simulink model "Vehicle_Model"  (R2018b)
settings: Solver=VariableStepAuto  StartTime=0  StopTime=60  FixedStep=0.0000001  RelTol=1e-10
undefined symbols (not defined in the file or in its folder): Initial
(part 4 of 4)

== matlab function Vehicle_Model/Subsystem3/MATLAB Function8 ==
  data: Fz input; Fxo output; kappa input; alpha input; gam input; Fzo input; Ro input; q_Bz1 input; q_Bz2 input; q_Bz3 input; q_Bz4 input; q_Bz5 input; q_Bz9 input; q_Bz10 input; q_Cz1 input; q_Dz1 input; q_Dz2 input; q_Dz3 input; q_Dz4 input; q_Dz6 input; q_Dz7 input; q_Dz8 input; q_Dz9 input; q_Ez1 input; q_Ez2 input; q_Ez3 input; q_Ez4 input; q_Ez5 input; q_Hz1 input; q_Hz2 input; q_Hz3 input; q_Hz4 input; p_Cy1 input; p_Dy1 input; p_Dy2 input; p_Dy3 input; p_Ey1 input; p_Ey2 input; p_Ey3 input; p_Ey4 input; p_Ky1 input; p_Ky2 input; p_Ky3 input; p_Hy1 input; p_Hy2 input; p_Hy3 input; p_Vy1 input; p_Vy2 input; p_Vy3 input; p_Vy4 input; p_Cx1 input; p_Dx1 input; p_Dx2 input; p_Ex1 input; p_Ex2 input; p_Ex3 input; p_Ex4 input; p_Kx1 input; p_Kx2 input; p_Kx3 input; p_Hx1 input; p_Hx2 input; p_Vx1 input; p_Vx2 input; car_mu_scaling input; run_info input; Fyo output; Mzo output
function [Fxo,Fyo,Mzo] = Pacejka_Tyre_Model(Fz,kappa,alpha,gam,Fzo,Ro,...
    q_Bz1,q_Bz2,q_Bz3,q_Bz4,q_Bz5,q_Bz9,q_Bz10,q_Cz1,q_Dz1,...
    q_Dz2,q_Dz3,q_Dz4,q_Dz6,q_Dz7,q_Dz8,q_Dz9,q_Ez1,q_Ez2,q_Ez3,q_Ez4,q_Ez5,...
    q_Hz1,q_Hz2,q_Hz3,q_Hz4,p_Cy1,p_Dy1,p_Dy2,p_Dy3,p_Ey1,p_Ey2,p_Ey3,...
    p_Ey4,p_Ky1,p_Ky2,p_Ky3,p_Hy1,p_Hy2,p_Hy3,p_Vy1,p_Vy2,p_Vy3,p_Vy4,...
    p_Cx1,p_Dx1,p_Dx2,p_Ex1,p_Ex2,p_Ex3,p_Ex4,p_Kx1,p_Kx2,p_Kx3,p_Hx1,...
    p_Hx2,p_Vx1,p_Vx2,car_mu_scaling,run_info)
% Pacejka '96 tyre model
%
% Inputs:
% Fz:       normal force (N)
% kappa:    slip ratio (% between -1 and 1) +ve is driving, -ve is braking
% alpha:    slip angle (rad) +ve alpha generates +ve Fyo
% gam:      inclanation angle./camber (rad) +ve indicates top of tyre tipped
%           right
% Outputs:
% Fxo:      Longitudinal force (N)
% Fyo:      Lateral force (N)
% Mzo:      Aligning moment (Nm)


%% tyre coefficients
% each different type of tyre holds different scaling coefficients, load 
% these here. Also loaded are unloaded tyre radius and nominal wheel load

% unpack the structure holding the coefficients
% Get the field names of the structure.
% fields = fieldnames(pacejka_coefs, '-full');
% 
% for ii = 1:length(fields)
%     thisField = fields{ii};
%     create_variable = sprintf('%s = pacejka_coefs.%s;', thisField, thisField);
%     eval(create_variable);
% end
% clear('ii', 'thisField');
% clear('fields', 'create_variable');

%% register track conditions
% scaling factors affected by wet/dry conditions
% if strcmp(run_info.track_conditions,'dry')
    lambda_mux = 1; % peak friction coefficient
    lambda_muy = 1; % peak friction coefficient
% elseif strcmp(run_info.track_conditions,'wet')
%     lambda_mux = 0.5; % peak friction coefficient
%     lambda_muy = 0.5; % peak friction coefficient
% else
%     fprintf('Track conditions incorrectly specified: dry condtitions used \n');
%     lambda_mux = 1; % peak friction coefficient
%     lambda_muy = 1; % peak friction coefficient
% end

% modify with user scaling factor
lambda_mux = lambda_mux*car_mu_scaling;
lambda_muy = lambda_muy*car_mu_scaling;

%% scaling factors
% default values for these values is 1 (except lambda_muV=0)
lambda_Fzo = 1; % nominal rated load
lambda_muV = 0; % with slip speed Vx decaying friction
lambda_Kx = 1; % brake slip stiffness
lambda_Ky = 1; % cornering stiffness
lambda_Cx = 1; % shape factor
lambda_Cy = 1; % shape factor
lambda_Ex = 1; % curvature factor
lambda_Ey = 1; % curvature factor
lambda_Hx = 1; % horizontal shift
lambda_Hy = 1; % horizontal shift
lambda_Vx = 1; % vertical shift
lambda_Vy = 1; % vertical shift
lambda_Kygam = 1; % camber force stiffness
lambda_Kzgam = 1; % camber torque stiffness
lambda_t = 1; % pneumatic trail
lambda_Mr = 1; % residual torque
lambda_ygam = 1;

if ~isrow(kappa) || ~isrow(alpha) || ~isrow(gam)
    kappa = transpose(kappa);
    alpha = transpose(alpha);
    gam = transpose(gam);
end

% for ii=1:length(Fz)
%     %% derived inputs
     dfz = (Fz-Fzo)/Fzo; % normalised change in vertical load
    
    %% longitudinal force (pure longitudinal slip)
    S_Vx = Fz*(p_Vx1+p_Vx2.*dfz).*lambda_Vx.*lambda_mux;
    S_Hx = (p_Hx1+p_Hx2.*dfz).*lambda_Hx;
    kappa_x = kappa + S_Hx;
    K_xk = Fz*(p_Kx1+p_Kx2.*dfz).*exp(-p_Kx3.*dfz).*lambda_Kx;
    E_x = (p_Ex1+p_Ex2.*dfz+p_Ex3.*dfz.^2).*(1-p_Ex4.*sign(kappa_x)).*lambda_Ex;
    mu_x = (p_Dx1+p_Dx2.*dfz).*lambda_mux;
    D_x = mu_x.*Fz;
    C_x = p_Cx1.*lambda_Cx;
    B_x = K_xk./(C_x.*D_x);
    Fxo = D_x.*sin(C_x.*atan(B_x.*kappa_x - E_x.*(B_x.*kappa_x-atan(B_x.*kappa_x)))) + S_Vx;
    
    %% lateral force (pure lateral slip)
    gam_y = gam.*lambda_ygam;
    C_y = p_Cy1.*lambda_Cy;
    mu_y = (p_Dy1+p_Dy2.*dfz).*(1-p_Dy3.*gam.^2).*lambda_muy;
    D_y = mu_y.*Fz;
    S_Hy = (p_Hy1+p_Hy2.*dfz+p_Hy3.*gam).*lambda_Hy;
    alpha_y = alpha + S_Hy;
    E_y = (p_Ey1+p_Ey2.*dfz).*(1-(p_Ey3+p_Ey4.*gam_y).*sign(alpha_y)).*lambda_Ey;
    K_ya = p_Ky1.*Fzo.*sin(2.*atan(Fz./(p_Ky2.*Fzo.*lambda_Fzo))).*(1-p_Ky3.*abs(gam)).*lambda_Fzo.*lambda_Ky;
    B_y = K_ya./(C_y.*D_y);
    S_Vy = Fz.*((p_Vy1+p_Vy2.*dfz)+(p_Vy3+p_Vy4.*dfz).*gam.*lambda_Vy.*lambda_Kygam);
    Fyo = D_y.*sin(C_y.*atan(B_y.*alpha_y - E_y.*(B_y.*alpha_y-atan(B_y.*alpha_y)))) + S_Vy;
    
    %% aligning torque (pure side slip)
    B_t = (q_Bz1+q_Bz2.*dfz+q_Bz3.*dfz.^2).*(1+q_Bz4.*gam.*q_Bz5.*abs(gam)).*lambda_Ky./lambda_muy;
    C_t = q_Cz1;
    D_t = (q_Dz1+q_Dz2.*dfz).*(1+q_Dz3.*gam+q_Dz4.*gam.^2).*Ro.*lambda_t./Fzo;
    S_Ht = q_Hz1+q_Hz2.*dfz+(q_Hz3+q_Hz4.*dfz).*gam;
    alpha_t = alpha + S_Ht;
    E_t = (q_Ez1+q_Ez2.*dfz+q_Ez3.*dfz.^2).*(1+(q_Ez4+q_Ez5.*gam).*atan(B_t.*C_t.*alpha_t));
    B_r = (q_Bz9.*lambda_Ky./lambda_muy+q_Bz10.*B_y.*C_y);
    D_r = Fz.*((q_Dz6+q_Dz7.*dfz)+(q_Dz8+q_Dz9.*dfz).*gam).*Ro.*lambda_muy.*lambda_Mr;
    S_Hf = S_Hy + S_Vy./K_ya;
    alpha_r = alpha + S_Hf;
    Mzr = D_r.*cos(atan(B_r.*alpha_r)).*cos(alpha);
    t = D_t.*cos(C_t.*atan(B_t.*alpha_t-E_t.*(B_t.*alpha_t-atan(B_t.*alpha_t)))).*cos(alpha);
    Mzo = -t.*Fyo + Mzr;
    
% end

== matlab function Vehicle_Model/Subsystem4/MATLAB Function ==
  data: x input; F_z output; xdot input; k input; c input
function F_z = fcn(x,xdot,k,c)

F_z = k * x + c * xdot;

== matlab function Vehicle_Model/Subsystem4/MATLAB Function8 ==
  data: Fz input; Fxo output; kappa input; alpha input; gam input; Fzo input; Ro input; q_Bz1 input; q_Bz2 input; q_Bz3 input; q_Bz4 input; q_Bz5 input; q_Bz9 input; q_Bz10 input; q_Cz1 input; q_Dz1 input; q_Dz2 input; q_Dz3 input; q_Dz4 input; q_Dz6 input; q_Dz7 input; q_Dz8 input; q_Dz9 input; q_Ez1 input; q_Ez2 input; q_Ez3 input; q_Ez4 input; q_Ez5 input; q_Hz1 input; q_Hz2 input; q_Hz3 input; q_Hz4 input; p_Cy1 input; p_Dy1 input; p_Dy2 input; p_Dy3 input; p_Ey1 input; p_Ey2 input; p_Ey3 input; p_Ey4 input; p_Ky1 input; p_Ky2 input; p_Ky3 input; p_Hy1 input; p_Hy2 input; p_Hy3 input; p_Vy1 input; p_Vy2 input; p_Vy3 input; p_Vy4 input; p_Cx1 input; p_Dx1 input; p_Dx2 input; p_Ex1 input; p_Ex2 input; p_Ex3 input; p_Ex4 input; p_Kx1 input; p_Kx2 input; p_Kx3 input; p_Hx1 input; p_Hx2 input; p_Vx1 input; p_Vx2 input; car_mu_scaling input; run_info input; Fyo output; Mzo output
function [Fxo,Fyo,Mzo] = Pacejka_Tyre_Model(Fz,kappa,alpha,gam,Fzo,Ro,...
    q_Bz1,q_Bz2,q_Bz3,q_Bz4,q_Bz5,q_Bz9,q_Bz10,q_Cz1,q_Dz1,...
    q_Dz2,q_Dz3,q_Dz4,q_Dz6,q_Dz7,q_Dz8,q_Dz9,q_Ez1,q_Ez2,q_Ez3,q_Ez4,q_Ez5,...
    q_Hz1,q_Hz2,q_Hz3,q_Hz4,p_Cy1,p_Dy1,p_Dy2,p_Dy3,p_Ey1,p_Ey2,p_Ey3,...
    p_Ey4,p_Ky1,p_Ky2,p_Ky3,p_Hy1,p_Hy2,p_Hy3,p_Vy1,p_Vy2,p_Vy3,p_Vy4,...
    p_Cx1,p_Dx1,p_Dx2,p_Ex1,p_Ex2,p_Ex3,p_Ex4,p_Kx1,p_Kx2,p_Kx3,p_Hx1,...
    p_Hx2,p_Vx1,p_Vx2,car_mu_scaling,run_info)
% Pacejka '96 tyre model
%
% Inputs:
% Fz:       normal force (N)
% kappa:    slip ratio (% between -1 and 1) +ve is driving, -ve is braking
% alpha:    slip angle (rad) +ve alpha generates +ve Fyo
% gam:      inclanation angle./camber (rad) +ve indicates top of tyre tipped
%           right
% Outputs:
% Fxo:      Longitudinal force (N)
% Fyo:      Lateral force (N)
% Mzo:      Aligning moment (Nm)


%% tyre coefficients
% each different type of tyre holds different scaling coefficients, load 
% these here. Also loaded are unloaded tyre radius and nominal wheel load

% unpack the structure holding the coefficients
% Get the field names of the structure.
% fields = fieldnames(pacejka_coefs, '-full');
% 
% for ii = 1:length(fields)
%     thisField = fields{ii};
%     create_variable = sprintf('%s = pacejka_coefs.%s;', thisField, thisField);
%     eval(create_variable);
% end
% clear('ii', 'thisField');
% clear('fields', 'create_variable');

%% register track conditions
% scaling factors affected by wet/dry conditions
% if strcmp(run_info.track_conditions,'dry')
    lambda_mux = 1; % peak friction coefficient
    lambda_muy = 1; % peak friction coefficient
% elseif strcmp(run_info.track_conditions,'wet')
%     lambda_mux = 0.5; % peak friction coefficient
%     lambda_muy = 0.5; % peak friction coefficient
% else
%     fprintf('Track conditions incorrectly specified: dry condtitions used \n');
%     lambda_mux = 1; % peak friction coefficient
%     lambda_muy = 1; % peak friction coefficient
% end

% modify with user scaling factor
lambda_mux = lambda_mux*car_mu_scaling;
lambda_muy = lambda_muy*car_mu_scaling;

%% scaling factors
% default values for these values is 1 (except lambda_muV=0)
lambda_Fzo = 1; % nominal rated load
lambda_muV = 0; % with slip speed Vx decaying friction
lambda_Kx = 1; % brake slip stiffness
lambda_Ky = 1; % cornering stiffness
lambda_Cx = 1; % shape factor
lambda_Cy = 1; % shape factor
lambda_Ex = 1; % curvature factor
lambda_Ey = 1; % curvature factor
lambda_Hx = 1; % horizontal shift
lambda_Hy = 1; % horizontal shift
lambda_Vx = 1; % vertical shift
lambda_Vy = 1; % vertical shift
lambda_Kygam = 1; % camber force stiffness
lambda_Kzgam = 1; % camber torque stiffness
lambda_t = 1; % pneumatic trail
lambda_Mr = 1; % residual torque
lambda_ygam = 1;

if ~isrow(kappa) || ~isrow(alpha) || ~isrow(gam)
    kappa = transpose(kappa);
    alpha = transpose(alpha);
    gam = transpose(gam);
end

% for ii=1:length(Fz)
%     %% derived inputs
     dfz = (Fz-Fzo)/Fzo; % normalised change in vertical load
    
    %% longitudinal force (pure longitudinal slip)
    S_Vx = Fz*(p_Vx1+p_Vx2.*dfz).*lambda_Vx.*lambda_mux;
    S_Hx = (p_Hx1+p_Hx2.*dfz).*lambda_Hx;
    kappa_x = kappa + S_Hx;
    K_xk = Fz*(p_Kx1+p_Kx2.*dfz).*exp(-p_Kx3.*dfz).*lambda_Kx;
    E_x = (p_Ex1+p_Ex2.*dfz+p_Ex3.*dfz.^2).*(1-p_Ex4.*sign(kappa_x)).*lambda_Ex;
    mu_x = (p_Dx1+p_Dx2.*dfz).*lambda_mux;
    D_x = mu_x.*Fz;
    C_x = p_Cx1.*lambda_Cx;
    B_x = K_xk./(C_x.*D_x);
    Fxo = D_x.*sin(C_x.*atan(B_x.*kappa_x - E_x.*(B_x.*kappa_x-atan(B_x.*kappa_x)))) + S_Vx;
    
    %% lateral force (pure lateral slip)
    gam_y = gam.*lambda_ygam;
    C_y = p_Cy1.*lambda_Cy;
    mu_y = (p_Dy1+p_Dy2.*dfz).*(1-p_Dy3.*gam.^2).*lambda_muy;
    D_y = mu_y.*Fz;
    S_Hy = (p_Hy1+p_Hy2.*dfz+p_Hy3.*gam).*lambda_Hy;
    alpha_y = alpha + S_Hy;
    E_y = (p_Ey1+p_Ey2.*dfz).*(1-(p_Ey3+p_Ey4.*gam_y).*sign(alpha_y)).*lambda_Ey;
    K_ya = p_Ky1.*Fzo.*sin(2.*atan(Fz./(p_Ky2.*Fzo.*lambda_Fzo))).*(1-p_Ky3.*abs(gam)).*lambda_Fzo.*lambda_Ky;
    B_y = K_ya./(C_y.*D_y);
    S_Vy = Fz.*((p_Vy1+p_Vy2.*dfz)+(p_Vy3+p_Vy4.*dfz).*gam.*lambda_Vy.*lambda_Kygam);
    Fyo = D_y.*sin(C_y.*atan(B_y.*alpha_y - E_y.*(B_y.*alpha_y-atan(B_y.*alpha_y)))) + S_Vy;
    
    %% aligning torque (pure side slip)
    B_t = (q_Bz1+q_Bz2.*dfz+q_Bz3.*dfz.^2).*(1+q_Bz4.*gam.*q_Bz5.*abs(gam)).*lambda_Ky./lambda_muy;
    C_t = q_Cz1;
    D_t = (q_Dz1+q_Dz2.*dfz).*(1+q_Dz3.*gam+q_Dz4.*gam.^2).*Ro.*lambda_t./Fzo;
    S_Ht = q_Hz1+q_Hz2.*dfz+(q_Hz3+q_Hz4.*dfz).*gam;
    alpha_t = alpha + S_Ht;
    E_t = (q_Ez1+q_Ez2.*dfz+q_Ez3.*dfz.^2).*(1+(q_Ez4+q_Ez5.*gam).*atan(B_t.*C_t.*alpha_t));
    B_r = (q_Bz9.*lambda_Ky./lambda_muy+q_Bz10.*B_y.*C_y);
    D_r = Fz.*((q_Dz6+q_Dz7.*dfz)+(q_Dz8+q_Dz9.*dfz).*gam).*Ro.*lambda_muy.*lambda_Mr;
    S_Hf = S_Hy + S_Vy./K_ya;
    alpha_r = alpha + S_Hf;
    Mzr = D_r.*cos(atan(B_r.*alpha_r)).*cos(alpha);
    t = D_t.*cos(C_t.*atan(B_t.*alpha_t-E_t.*(B_t.*alpha_t-atan(B_t.*alpha_t)))).*cos(alpha);
    Mzo = -t.*Fyo + Mzr;
    
% end

== matlab function Vehicle_Model/Chassis Vertical 8DOF/MATLAB Function ==
  data: initial output
function initial = Chassis8_Initial()
% Initial Conditions
z_c = -0.25;
y_thetaC = 0;
x_thetaCF = 0;
x_thetaCR = 0;
x_WFR = -0.04;
x_WFL = -0.04;
x_WRR = -0.04;
x_WRL = -0.04;
zdot_c = 0;
ydot_thetaC = 0;
xdot_thetaCF = 0;
xdot_thetaCR = 0;
xdot_WFR = 0;
xdot_WFL = 0;
xdot_WRR = 0;
xdot_WRL = 0;

initial = [z_c, zdot_c,...
    y_thetaC, ydot_thetaC,...
    x_thetaCF, xdot_thetaCF,...
    x_thetaCR, xdot_thetaCR,...
    x_WFR, xdot_WFR,...
    x_WFL, xdot_WFL,...
    x_WRR, xdot_WRR,...
    x_WRL, xdot_WRL];

== matlab function Vehicle_Model/MATLAB Function26 ==
  data: t input; S_FR output; S_FL output; S_RR output; S_RL output
function [S_FR,S_FL,S_RR,S_RL] = Steering_Angles(t)

S_FR = 0.5 * sin(t);
S_FL = 0.5 * sin(t);
S_RR = 0;
S_RL = 0;
